simulink model "PID"  (R2021a)
settings: Solver=VariableStepAuto  StartTime=0.0  StopTime=10.0  RelTol=1e-3
libraries: arduinolib x8, simulink x1, realtime_examples_misc x1
settings Model: Creator=temis  LastModifiedBy=temis

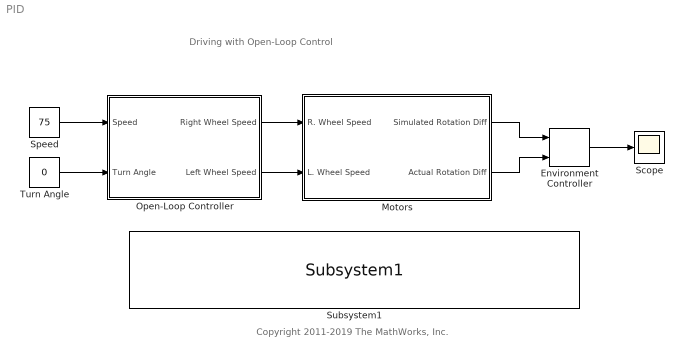
== system PID ==
  note: Driving with Open-Loop Control
  note: Copyright 2011-2019 The MathWorks, Inc.
  Environment Controller : simulink/Signal Routing/Environment Controller
      settings: SourceProductBaseCode=SL
  Motors : Subsystem  VariantControl=DoSim
  Open-Loop Controller : Subsystem
  Scope : Scope
  Speed : Constant  Value=75  OutMin=0  OutMax=100  OutDataTypeStr=single  SampleTime=0.001
  Subsystem1 : realtime_examples_misc/Subsystem1  SystemSampleTime=-1  VariantActivationTime=update diagram  Latency=0  AutoFrameSizeCalculation=off
      settings: SourceProductBaseCode=SL
  Turn Angle : Constant  Value=0  OutMin=-50  OutMax=50  OutDataTypeStr=single  SampleTime=0.001
  wires:
  Speed/1 -> Open-Loop Controller/1(Speed)
  Turn Angle/1 -> Open-Loop Controller/2(Turn Angle)
  Open-Loop Controller/1(Right Wheel Speed) -> Motors/1(R. Wheel Speed)
  Open-Loop Controller/2(Left Wheel Speed) -> Motors/2(L. Wheel Speed)
  Environment Controller/1 -> Scope/1
  Motors/1(Simulated Rotation Diff) -> Environment Controller/1
  Motors/2(Actual Rotation Diff) -> Environment Controller/2

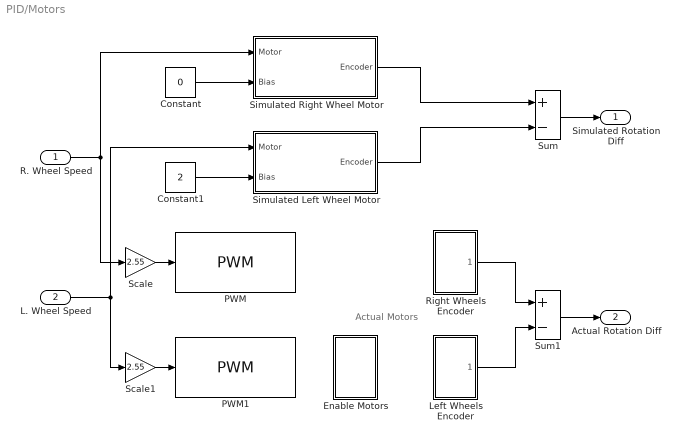
== system PID/Motors ==
  note: Actual
      | Motors
  R. Wheel Speed : Inport
  L. Wheel Speed : Inport  Port=2
  Constant : Constant  Value=0  OutDataTypeStr=single
  Constant1 : Constant  Value=2  OutDataTypeStr=single
  Enable Motors : Subsystem
  Left Wheels Encoder : Subsystem
  PWM : arduinolib/PWM  pinNumber=10  frequencyType=Default  desiredFrequency=490.2  achievableFrequency=490.2
  PWM1 : arduinolib/PWM  pinNumber=11  frequencyType=Default  desiredFrequency=490.2  achievableFrequency=490.2
  Right Wheels Encoder : Subsystem
  Scale : Gain  Gain=2.55
  Scale1 : Gain  Gain=2.55
  Simulated Left Wheel Motor : Subsystem
  Simulated Right Wheel Motor : Subsystem
  Sum : Sum  Inputs=+-  OutDataTypeStr=Inherit: Same as first input
  Sum1 : Sum  Inputs=+-  OutDataTypeStr=Inherit: Same as first input
  Simulated Rotation Diff : Outport  VectorParamsAs1DForOutWhenUnconnected=off
  Actual Rotation Diff : Outport  Port=2  VectorParamsAs1DForOutWhenUnconnected=off
  wires:
  Sum1/1 -> Actual Rotation Diff/1
  Sum/1 -> Simulated Rotation Diff/1
  Simulated Left Wheel Motor/1(Encoder) -> Sum/2
  Simulated Right Wheel Motor/1(Encoder) -> Sum/1
  R. Wheel Speed/1 -> Simulated Right Wheel Motor/1(Motor), Scale/1
  L. Wheel Speed/1 -> Simulated Left Wheel Motor/1(Motor), Scale1/1
  Constant/1 -> Simulated Right Wheel Motor/2(Bias)
  Constant1/1 -> Simulated Left Wheel Motor/2(Bias)
  Left Wheels Encoder/1(Encoder) -> Sum1/2
  Right Wheels Encoder/1(Encoder) -> Sum1/1
  Scale/1 -> PWM/1
  Scale1/1 -> PWM1/1

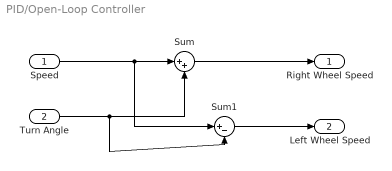
== system PID/Open-Loop Controller ==
  Speed : Inport
  Turn Angle : Inport  Port=2
  Sum : Sum  Inputs=|++  OutDataTypeStr=Inherit: Same as first input
  Sum1 : Sum  Inputs=|+-  OutDataTypeStr=Inherit: Same as first input
  Right Wheel Speed : Outport  VectorParamsAs1DForOutWhenUnconnected=off
  Left Wheel Speed : Outport  Port=2  VectorParamsAs1DForOutWhenUnconnected=off
  wires:
  Sum1/1 -> Left Wheel Speed/1
  Sum/1 -> Right Wheel Speed/1
  Turn Angle/1 -> Sum1/2, Sum/2
  Speed/1 -> Sum1/1, Sum/1

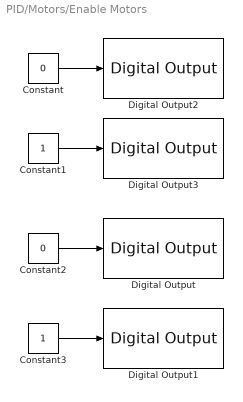
== system PID/Motors/Enable Motors ==
  Constant : Constant  Value=0  OutDataTypeStr=boolean
  Constant1 : Constant  OutDataTypeStr=boolean
  Constant2 : Constant  Value=0  OutDataTypeStr=boolean
  Constant3 : Constant  OutDataTypeStr=boolean
  Digital Output : arduinolib/Digital Output  pinNumber=2  Direction=output  blockPlatform=arduino
  Digital Output1 : arduinolib/Digital Output  pinNumber=3  Direction=output  blockPlatform=arduino
  Digital Output2 : arduinolib/Digital Output  pinNumber=4  Direction=output  blockPlatform=arduino
  Digital Output3 : arduinolib/Digital Output  pinNumber=5  Direction=output  blockPlatform=arduino
  wires:
  Constant1/1 -> Digital Output3/1
  Constant/1 -> Digital Output2/1
  Constant2/1 -> Digital Output/1
  Constant3/1 -> Digital Output1/1

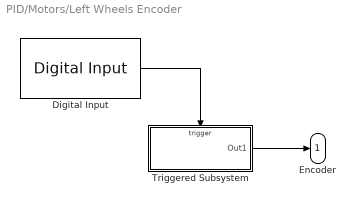
== system PID/Motors/Left Wheels Encoder ==
  Digital Input : arduinolib/Digital Input  pinNumber=9  mode=Default  Direction=input  SampleTime=0.001  blockPlatform=arduino
  Triggered Subsystem : Subsystem  TreatAsAtomicUnit=on
  Encoder : Outport  VectorParamsAs1DForOutWhenUnconnected=off
  wires:
  Digital Input/1 -> Triggered Subsystem/Trigger
  Triggered Subsystem/1(Out1) -> Encoder/1

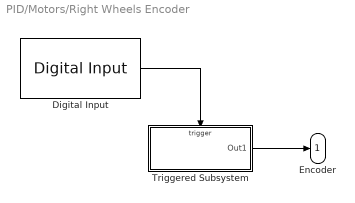
== system PID/Motors/Right Wheels Encoder ==
  Digital Input : arduinolib/Digital Input  pinNumber=8  mode=Default  Direction=input  SampleTime=0.001  blockPlatform=arduino
  Triggered Subsystem : Subsystem  TreatAsAtomicUnit=on
  Encoder : Outport  VectorParamsAs1DForOutWhenUnconnected=off
  wires:
  Triggered Subsystem/1(Out1) -> Encoder/1
  Digital Input/1 -> Triggered Subsystem/Trigger

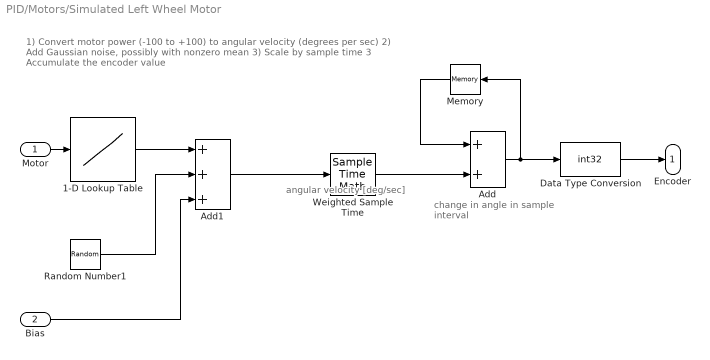
== system PID/Motors/Simulated Left Wheel Motor ==
  note: change in angle
      | in sample interval
  note: angular velocity
      | [deg/sec]
  note: 1) Convert motor power (-100 to +100) to angular velocity (degrees per sec)
      | 2) Add Gaussian noise, possibly with nonzero mean
      | 3) Scale by sample time
      | 3 Accumulate the encoder value
  Motor : Inport
  Bias : Inport  Port=2
  1-D Lookup Table : Lookup_n-D  NumberOfTableDimensions=1  BreakpointsForDimension1=[-100 0 100]  Table=[-360 0 360]  ExtrapMethod=Clip  UseLastTableValue=on  RndMeth=Simplest  InputSameDT=on
  Add : Sum  OutDataTypeStr=Inherit: Same as first input
  Add1 : Sum  Inputs=+++  OutDataTypeStr=single
  Data Type Conversion : DataTypeConversion  OutDataTypeStr=int32
  Memory : Memory  InheritSampleTime=on  LinearizeAsDelay=on
  Random Number1 : RandomNumber  Variance=5  Seed=randi(1000)
  Weighted Sample Time : SampleTimeMath  TsampMathOp=*
  Encoder : Outport  VectorParamsAs1DForOutWhenUnconnected=off
  wires:
  Data Type Conversion/1 -> Encoder/1
  Bias/1 -> Add1/3
  Weighted Sample Time/1 -> Add/2
  Add/1 -> Data Type Conversion/1, Memory/1
  Memory/1 -> Add/1
  Add1/1 -> Weighted Sample Time/1
  Motor/1 -> 1-D Lookup Table/1
  Random Number1/1 -> Add1/2
  1-D Lookup Table/1 -> Add1/1

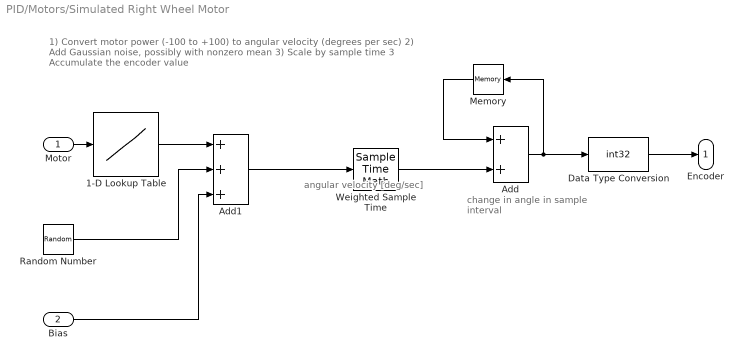
== system PID/Motors/Simulated Right Wheel Motor ==
  note: 1) Convert motor power (-100 to +100) to angular velocity (degrees per sec)
      | 2) Add Gaussian noise, possibly with nonzero mean
      | 3) Scale by sample time
      | 3 Accumulate the encoder value
  note: angular velocity
      |  [deg/sec]
  note: change in angle
      | in sample interval
  Motor : Inport
  Bias : Inport  Port=2
  1-D Lookup Table : Lookup_n-D  NumberOfTableDimensions=1  BreakpointsForDimension1=[-100 0 100]  Table=[-360 0 360]  ExtrapMethod=Clip  UseLastTableValue=on  RndMeth=Simplest  InputSameDT=on
  Add : Sum  AccumDataTypeStr=single  OutDataTypeStr=single
  Add1 : Sum  Inputs=+++  OutDataTypeStr=single
  Data Type Conversion : DataTypeConversion  OutDataTypeStr=int32
  Memory : Memory  InheritSampleTime=on  LinearizeAsDelay=on
  Random Number : RandomNumber  Variance=5  Seed=randi(1000)
  Weighted Sample Time : SampleTimeMath  TsampMathOp=*
  Encoder : Outport  VectorParamsAs1DForOutWhenUnconnected=off
  wires:
  Data Type Conversion/1 -> Encoder/1
  1-D Lookup Table/1 -> Add1/1
  Random Number/1 -> Add1/2
  Motor/1 -> 1-D Lookup Table/1
  Memory/1 -> Add/1
  Add/1 -> Data Type Conversion/1, Memory/1
  Weighted Sample Time/1 -> Add/2
  Bias/1 -> Add1/3
  Add1/1 -> Weighted Sample Time/1

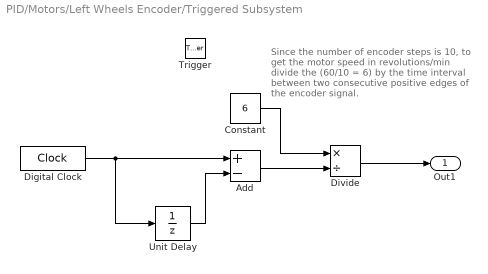
== system PID/Motors/Left Wheels Encoder/Triggered Subsystem ==
  note: Since the number of encoder steps is 10,
      | to get the motor speed in revolutions/min
      | divide the (60/10 = 6) by the time interval
      | between two consecutive positive edges
      | of the encoder signal.
  Trigger : TriggerPort  VariantControl=Variant
  Add : Sum  Inputs=+-
  Constant : Constant  Value=6
  Digital Clock : DigitalClock  SampleTime=-1
  Divide : Product  Inputs=*/  OutDataTypeStr=int32
  Unit Delay : UnitDelay  SampleTime=-1  HasFrameUpgradeWarning=on
  Out1 : Outport  VectorParamsAs1DForOutWhenUnconnected=off
  wires:
  Constant/1 -> Divide/1
  Divide/1 -> Out1/1
  Add/1 -> Divide/2
  Unit Delay/1 -> Add/2
  Digital Clock/1 -> Unit Delay/1, Add/1

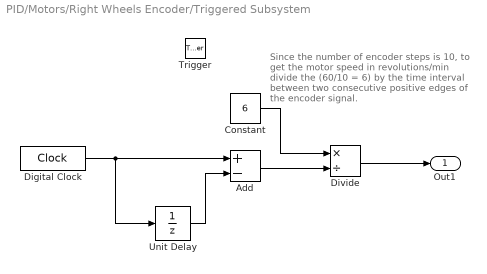
== system PID/Motors/Right Wheels Encoder/Triggered Subsystem ==
  note: Since the number of encoder steps is 10,
      | to get the motor speed in revolutions/min
      | divide the (60/10 = 6) by the time interval
      | between two consecutive positive edges
      | of the encoder signal.
  Trigger : TriggerPort  VariantControl=Variant
  Add : Sum  Inputs=+-
  Constant : Constant  Value=6
  Digital Clock : DigitalClock  SampleTime=-1
  Divide : Product  Inputs=*/  OutDataTypeStr=int32
  Unit Delay : UnitDelay  SampleTime=-1  HasFrameUpgradeWarning=on
  Out1 : Outport  VectorParamsAs1DForOutWhenUnconnected=off
  wires:
  Digital Clock/1 -> Add/1, Unit Delay/1
  Unit Delay/1 -> Add/2
  Add/1 -> Divide/2
  Divide/1 -> Out1/1
  Constant/1 -> Divide/1
